simulink model "Single_phase_Dual_Converter_R_Load"  (R2023b)
settings: Solver=VariableStepAuto  StartTime=0.0  StopTime=2.0  RelTol=1e-3
libraries: spsMosfetLib x4, spsThyristorLib x4, spsVoltageMeasurementLib x3, spsSeriesRLCBranchLib x2, spsACVoltageSourceLib x1, sps_lib x1
settings Model: Creator=HP  LastModifiedBy=HP

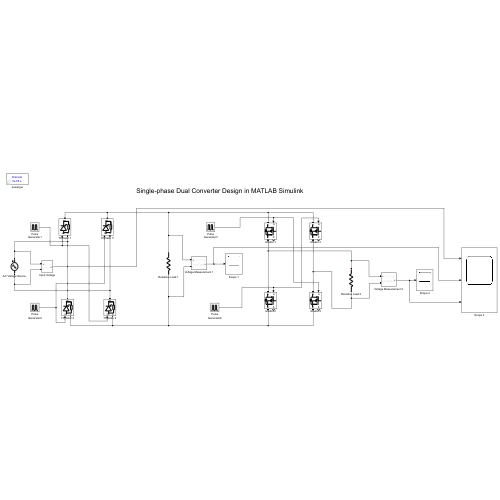
[thumbnail: Simulink's stored preview of the top-level diagram]
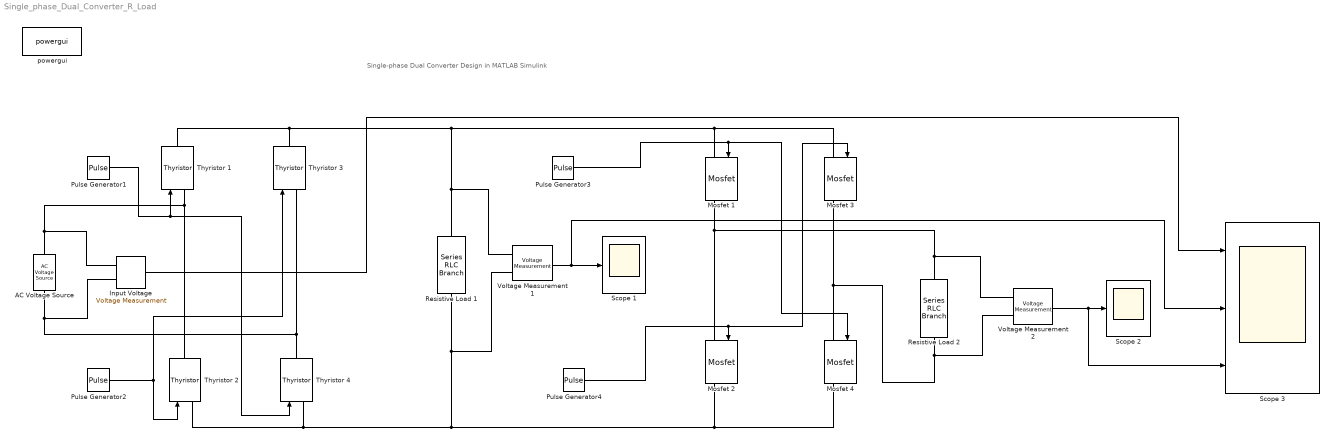
== system Single_phase_Dual_Converter_R_Load ==
  note: Single-phase Dual Converter Design in MATLAB Simulink
  AC Voltage Source : spsACVoltageSourceLib/AC Voltage Source  Amplitude=325.15  Phase=0  Frequency=50  SampleTime=0  Measurements=None  BusType=swing  Pref=10e3  Qref=0  Qmin=-inf  Qmax=+inf
  Input Voltage : spsVoltageMeasurementLib/Voltage Measurement  PhasorSimulation=off  OutputType=Complex  PSBequivalent=0
  Mosfet {1..4} (4 alike) : spsMosfetLib/Mosfet  Ron=0.1  Lon=0  Rd=0.01  Vfd=0  IC=0  Rs=1e5  Cs=inf  Measurements=on
  Pulse Generator1 : DiscretePulseGenerator  PulseType=Time based  Period=0.02  PulseWidth=50
  Pulse Generator2 : DiscretePulseGenerator  PulseType=Time based  Period=0.02  PulseWidth=50  PhaseDelay=0.01
  Pulse Generator3 : DiscretePulseGenerator  PulseType=Time based  Period=0.02  PulseWidth=50
  Pulse Generator4 : DiscretePulseGenerator  PulseType=Time based  Period=0.02  PulseWidth=50  PhaseDelay=0.01
  Resistive Load 1 : spsSeriesRLCBranchLib/Series RLC Branch  LConnTagsString=__new0  RConnTagsString=__new0  BranchType=R  Resistance=300  Inductance=1e-3  SetiL0=off  InitialCurrent=0  Capacitance=1e-6  Setx0=off  InitialVoltage=0  Measurements=None
  Resistive Load 2 : spsSeriesRLCBranchLib/Series RLC Branch  LConnTagsString=__new0  RConnTagsString=__new0  BranchType=R  Resistance=300  Inductance=1e-3  SetiL0=off  InitialCurrent=0  Capacitance=1e-6  Setx0=off  InitialVoltage=0  Measurements=None
  Scope 1 : Scope
  Scope 2 : Scope
  Scope 3 : Scope  NumInputPorts=3
  Thyristor {1..4} (4 alike) : spsThyristorLib/Thyristor  Ron=0.001  Lon=0  Vf=0.8  IC=0  Rs=500  Cs=250e-9  Measurements=off
  Voltage Measurement 1 : spsVoltageMeasurementLib/Voltage Measurement  PhasorSimulation=off  OutputType=Complex  PSBequivalent=0
  Voltage Measurement 2 : spsVoltageMeasurementLib/Voltage Measurement  PhasorSimulation=off  OutputType=Complex  PSBequivalent=0
  powergui : sps_lib/powergui  Priority=1  SimulationMode=Discrete  SampleTime=50e-6  frequency=60  Iterations=50  frequencyindice=50  Pbase=100e6  ErrMax=1e-4  UnitsV=kV  UnitsW=MW  buscounter=0  FunctionMessages=off  echomessages=off  EnableUseOfTLC=off  CurrentSourceSwitches=off  DisableSnubberDevices=off  DisableRonSwitches=off  DisableVfSwitches=off  DisplayEquations=off  AutomaticDiscreteSolvers=off  SolverType=Tustin/Backward Euler (TBE)  Interpol=off  ExternalGateDelay=off  methode=off  Ts=100  x0status=blocks  SPID=on  SwTol=0  HookPort=off  NonlinearTolerance=1e-4  nMaxIteration=100  ContinueOnMaxIteration=off  RestoreLinks=warning  ResistiveCurrentMeasurement=off  Frange=[0:2:500]  Ylog=off  Xlog=on  ShowGrid=off  save=off  variable=ZData  structure=0  ZoomFFT=off  StartTime=0.0  cycles=1  DisplayStyle=1  fundamental=60  FreqAxis=off  MaxFrequency=1000  frequencyindicesteady=1  RmsSteady=1  display=off
  wires:
  Pulse Generator1/1 -> Thyristor 4/1, Thyristor 1/1
  Voltage Measurement 1/1 -> Scope 3/2, Scope 1/1
  Pulse Generator3/1 -> Mosfet 4/1, Mosfet 1/1
  Pulse Generator4/1 -> Mosfet 3/1, Mosfet 2/1
  Voltage Measurement 2/1 -> Scope 3/3, Scope 2/1
  Input Voltage/1 -> Scope 3/1
  Pulse Generator2/1 -> Thyristor 2/1, Thyristor 3/1
  connections:
  Thyristor 2/RConn1 -- AC Voltage Source/RConn1 -- Input Voltage/LConn1 -- Thyristor 1/LConn1
  Thyristor 4/RConn1 -- Thyristor 3/LConn1 -- AC Voltage Source/LConn1 -- Input Voltage/LConn2
  Thyristor 2/LConn1 -- Mosfet 4/RConn1 -- Mosfet 2/RConn1 -- Resistive Load 1/RConn1 -- Voltage Measurement 1/LConn2 -- Thyristor 4/LConn1
  Mosfet 1/RConn1 -- Voltage Measurement 2/LConn1 -- Resistive Load 2/LConn1 -- Mosfet 2/LConn1
  Mosfet 4/LConn1 -- Voltage Measurement 2/LConn2 -- Resistive Load 2/RConn1 -- Mosfet 3/RConn1
  Mosfet 1/LConn1 -- Thyristor 1/RConn1 -- Thyristor 3/RConn1 -- Resistive Load 1/LConn1 -- Voltage Measurement 1/LConn1 -- Mosfet 3/LConn1
